simulink subsystem "PvtSubSys_LONC"  (R2020b)
settings: Solver=VariableStepAuto  StartTime=0.0  StopTime=10.0  RelTol=1e-3
undefined symbols (not defined in the file): P_Global_TireRadius_m, P_Global_Weight_N, P_LongCtrl_VLC_fRollCoef, P_LongCtrl_VLC_WindArea, P_LongCtrl_VLCaccelMinHoldXAxis, P_LongCtrl_VLCaccelMinHoldYAxis, P_LongCtrl_VLCaXCDeadZoneProp_Y, P_LongCtrl_VLCaXCKiCtrlDevChar_Y, P_LongCtrl_VLCaxCtrlDevDeadZoneChar_Y, P_LongCtrl_VLCaxCtrlDevEC2DCMax, P_LongCtrl_VLCaxCtrlDevFastQuitDCMode, P_LongCtrl_VLCaxCtrlDevThresAddEC2DC, P_LongCtrl_VLCaxCtrlDevTresAddDC2EC, P_LongCtrl_VLCAxTarDtThreEnableI, P_LongCtrl_VLCaxvRoadSlopeDC4CharXAxis, P_LongCtrl_VLCaxvRoadSlopeDC4CharYAxis, P_LongCtrl_VLCAxvTracMinDC1FullFillXAxis, P_LongCtrl_VLCAxvTracMinDC1FullFillYAxis, P_LongCtrl_VLCcoefFXAxis, P_LongCtrl_VLCcoefFYAxis, P_LongCtrl_VLCcoefIFadeOut1Calc, P_LongCtrl_VLCcoefIFadeOut1Condition, P_LongCtrl_VLCcoefIFadeOut2Calc, P_LongCtrl_VLCcoefIFadeOut2Condition, P_LongCtrl_VLCcoefIFadeOut3Calc, P_LongCtrl_VLCcoefIFadeOut3Condition, P_LongCtrl_VLCCounterAxvTracMinTimeout, P_LongCtrl_VLCCounterDC2ECTorqDelay, P_LongCtrl_VLCCounterDrvOff2EC, P_LongCtrl_VLCdaxTarEC2DCMax, P_LongCtrl_VLCdriveOffAxUpLimXAxix, P_LongCtrl_VLCdriveOffAxUpLimYAxix, P_LongCtrl_VLCDtAxvRef2UpperBandDC5, P_LongCtrl_VLCIACompensionNeg, P_LongCtrl_VLCIACompensionPos, P_LongCtrl_VLCjerkHoldXAxis, P_LongCtrl_VLCjerkHoldYAxis, P_LongCtrl_VLCki, P_LongCtrl_VLCkp, P_LongCtrl_VLCks, P_LongCtrl_VLCTorqDiffThreAxvTracMinTimeout, P_LongCtrl_VLCTrTatioMax, P_LongCtrl_VLCTrTatioMin, P_LongCtrl_VLCVlcAccThresAxvTracMinTimeout
libraries: simulink x32
(part 1 of 2)
settings Model: Creator=GW00133806  LastModifiedBy=GW00119710

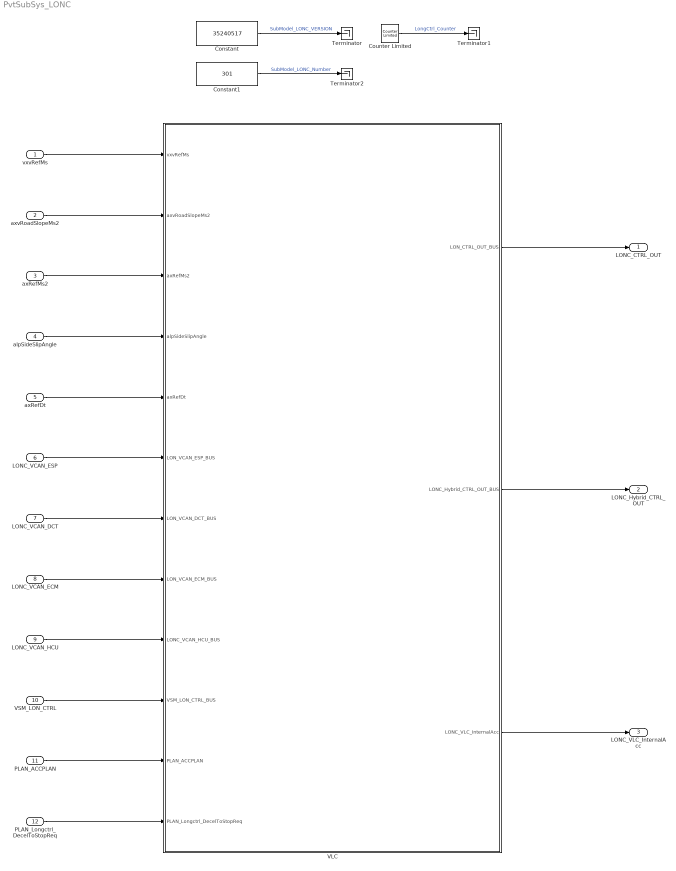
== system PvtSubSys_LONC ==
  vxvRefMs : Inport  OutDataTypeStr=single  PortDimensions=1  BusOutputAsStruct=on
  axvRoadSlopeMs2 : Inport  Port=2  OutDataTypeStr=single  PortDimensions=1  BusOutputAsStruct=on
  axRefMs2 : Inport  Port=3  OutDataTypeStr=single  PortDimensions=1  BusOutputAsStruct=on
  alpSideSlipAngle : Inport  Port=4  OutDataTypeStr=single  PortDimensions=1  BusOutputAsStruct=on
  axRefDt : Inport  Port=5  OutDataTypeStr=single  PortDimensions=1  BusOutputAsStruct=on
  LONC_VCAN_ESP : Inport  Port=6  OutDataTypeStr=Bus: VCAN_ESP_MSG_BUS  PortDimensions=1  BusOutputAsStruct=on
  LONC_VCAN_DCT : Inport  Port=7  OutDataTypeStr=Bus: VCAN_DCT_MSG_BUS  PortDimensions=1  BusOutputAsStruct=on
  LONC_VCAN_ECM : Inport  Port=8  OutDataTypeStr=Bus: VCAN_ECM_MSG_BUS  PortDimensions=1  BusOutputAsStruct=on
  LONC_VCAN_HCU : Inport  Port=9  OutDataTypeStr=Bus: VCAN_HCU_MSG_BUS  PortDimensions=1  BusOutputAsStruct=on
  VSM_LON_CTRL : Inport  Port=10  OutDataTypeStr=Bus: VSM_LON_CTRL_BUS  PortDimensions=1  BusOutputAsStruct=on
  PLAN_ACCPLAN : Inport  Port=11  OutDataTypeStr=Bus: PLAN_ACCPLAN_BUS
  PLAN_Longctrl_DecelToStopReq : Inport  Port=12  OutDataTypeStr=boolean  PortDimensions=1  BusOutputAsStruct=on
  Constant : Constant  Value=35240517  OutDataTypeStr=uint32
  Constant1 : Constant  Value=301  OutDataTypeStr=uint32
  Counter Limited : simulink/Sources/Counter Limited  uplimit=15  tsamp=-1
  Terminator : Terminator
  Terminator1 : Terminator
  Terminator2 : Terminator
  VLC : Subsystem
  LONC_CTRL_OUT : Outport  OutDataTypeStr=Bus: LONC_CTRL_OUT_BUS  PortDimensions=1  BusOutputAsStruct=on
  LONC_Hybrid_CTRL_OUT : Outport  Port=2  OutDataTypeStr=Bus: LONC_Hybrid_CTRL_OUT_BUS  PortDimensions=1  BusOutputAsStruct=on
  LONC_VLC_InternalAcc : Outport  Port=3  OutDataTypeStr=single
  wires:
  axRefDt/1 -> VLC/5(axRefDt)
  LONC_VCAN_ESP/1 -> VLC/6(LON_VCAN_ESP_BUS)
  PLAN_Longctrl_DecelToStopReq/1 -> VLC/12(PLAN_Longctrl_DecelToStopReq)
  alpSideSlipAngle/1 -> VLC/4(alpSideSlipAngle)
  vxvRefMs/1 -> VLC/1(vxvRefMs)
  Counter Limited/1 -> Terminator1/1  "LongCtrl_Counter"
  axRefMs2/1 -> VLC/3(axRefMs2)
  axvRoadSlopeMs2/1 -> VLC/2(axvRoadSlopeMs2)
  VLC/1(LON_CTRL_OUT_BUS) -> LONC_CTRL_OUT/1
  VSM_LON_CTRL/1 -> VLC/10(VSM_LON_CTRL_BUS)
  PLAN_ACCPLAN/1 -> VLC/11(PLAN_ACCPLAN)
  VLC/2(LONC_Hybrid_CTRL_OUT_BUS) -> LONC_Hybrid_CTRL_OUT/1
  LONC_VCAN_ECM/1 -> VLC/8(LON_VCAN_ECM_BUS)
  VLC/3(LONC_VLC_InternalAcc) -> LONC_VLC_InternalAcc/1
  LONC_VCAN_DCT/1 -> VLC/7(LON_VCAN_DCT_BUS)
  LONC_VCAN_HCU/1 -> VLC/9(LONC_VCAN_HCU_BUS)
  Constant/1 -> Terminator/1  "SubModel_LONC_VERSION"
  Constant1/1 -> Terminator2/1  "SubModel_LONC_Number"

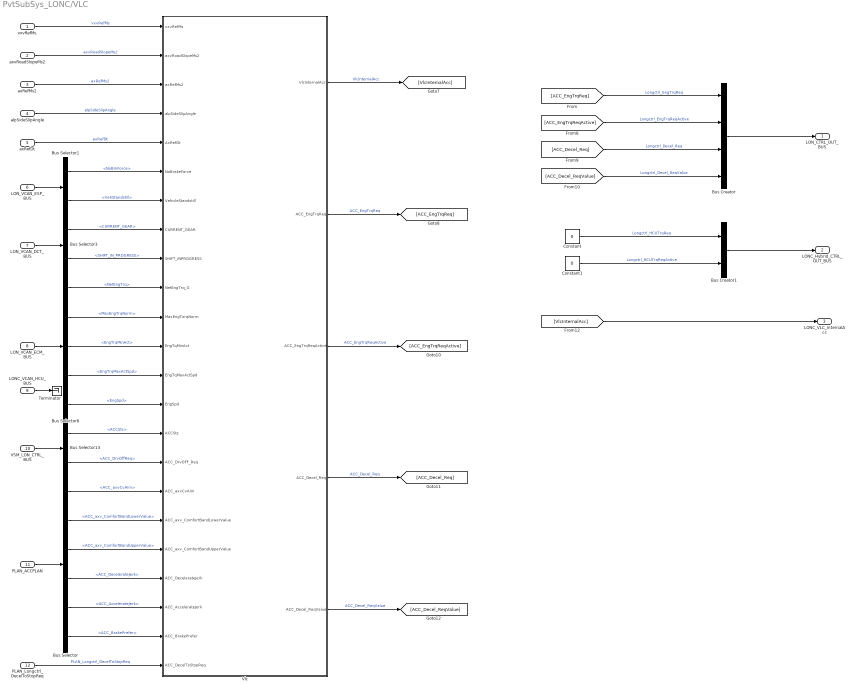
== system PvtSubSys_LONC/VLC ==
  vxvRefMs : Inport
  axvRoadSlopeMs2 : Inport  Port=2
  axRefMs2 : Inport  Port=3
  alpSideSlipAngle : Inport  Port=4
  axRefDt : Inport  Port=5
  LON_VCAN_ESP_BUS : Inport  Port=6  OutDataTypeStr=Bus: VCAN_ESP_MSG_BUS
  LON_VCAN_DCT_BUS : Inport  Port=7  OutDataTypeStr=Bus: VCAN_DCT_MSG_BUS
  LON_VCAN_ECM_BUS : Inport  Port=8  OutDataTypeStr=Bus: VCAN_ECM_MSG_BUS
  LONC_VCAN_HCU_BUS : Inport  Port=9  OutDataTypeStr=Bus: VCAN_HCU_MSG_BUS
  VSM_LON_CTRL_BUS : Inport  Port=10  OutDataTypeStr=Bus: VSM_LON_CTRL_BUS
  PLAN_ACCPLAN : Inport  Port=11  OutDataTypeStr=Bus: PLAN_ACCPLAN_BUS
  PLAN_Longctrl_DecelToStopReq : Inport  Port=12  OutDataTypeStr=boolean
  Bus Creator : BusCreator  Inputs=4  OutDataTypeStr=Bus: LONC_CTRL_OUT_BUS  NonVirtualBus=on
  Bus Creator1 : BusCreator  Inputs=2  OutDataTypeStr=Bus: LONC_Hybrid_CTRL_OUT_BUS  NonVirtualBus=on
  Bus Selector : BusSelector  OutputSignals=ACC_axvCvAim,ACC_axv_ComfortBandLowerValue,ACC_axv_ComfortBandUpperValue,ACC_DecelerateJerk,ACC_AccelerateJerk,ACC_BrakePrefer
  Bus Selector1 : BusSelector  OutputSignals=NoBrkForce,VehStandstill
  Bus Selector13 : BusSelector  OutputSignals=ACCSts,ACC_DrvOffReq
  Bus Selector3 : BusSelector  OutputSignals=CURRENT_GEAR,SHIFT_IN_PROGRESS
  Bus Selector6 : BusSelector  OutputSignals=NetEngTrq,MaxEngTrqNorm,EngTrqMinAct,EngTrqMaxActSpd,EngSpd
  Constant : Constant  Value=0  OutDataTypeStr=single
  Constant1 : Constant  Value=0  OutDataTypeStr=boolean
  Terminator : Terminator
  Vlc : Subsystem  TreatAsAtomicUnit=on
  LON_CTRL_OUT_BUS : Outport  OutDataTypeStr=Bus: LONC_CTRL_OUT_BUS
  LONC_Hybrid_CTRL_OUT_BUS : Outport  Port=2  OutDataTypeStr=Bus: LONC_Hybrid_CTRL_OUT_BUS
  LONC_VLC_InternalAcc : Outport  Port=3  OutDataTypeStr=single
  wires:
  LONC_VCAN_HCU_BUS/1 -> Terminator/1
  Constant/1 -> Bus Creator1/1  "Longctrl_HCUTrqReq"
  Constant1/1 -> Bus Creator1/2  "Longctrl_HCUTrqReqActive"
  Bus Creator1/1 -> LONC_Hybrid_CTRL_OUT_BUS/1
  PLAN_Longctrl_DecelToStopReq/1 -> Vlc/23(ACC_DecelToStopReq)  "PLAN_Longctrl_DecelToStopReq"
  [VlcInternalAcc] -> LONC_VLC_InternalAcc/1
  Bus Selector/1 -> Vlc/17(ACC_axvCvAim)  "<ACC_axvCvAim>"
  Bus Selector/6 -> Vlc/22(ACC_BrakePrefer)  "<ACC_BrakePrefer>"
  Bus Selector/2 -> Vlc/18(ACC_axv_ComfortBandLowerValue)  "<ACC_axv_ComfortBandLowerValue>"
  Bus Selector/3 -> Vlc/19(ACC_axv_ComfortBandUpperValue)  "<ACC_axv_ComfortBandUpperValue>"
  Bus Selector/5 -> Vlc/21(ACC_AccelerateJerk)  "<ACC_AccelerateJerk>"
  Bus Selector/4 -> Vlc/20(ACC_DecelerateJerk)  "<ACC_DecelerateJerk>"
  PLAN_ACCPLAN/1 -> Bus Selector/1
  alpSideSlipAngle/1 -> Vlc/4(alpSideSlipAngle)  "alpSideSlipAngle"
  Bus Selector13/2 -> Vlc/16(ACC_DrvOFF_Req)  "<ACC_DrvOffReq>"
  Bus Selector13/1 -> Vlc/15(ACCSts)  "<ACCSts>"
  VSM_LON_CTRL_BUS/1 -> Bus Selector13/1
  Bus Selector6/5 -> Vlc/14(EngSpd)  "<EngSpd>"
  Bus Selector6/4 -> Vlc/13(EngTqMaxActSpd)  "<EngTrqMaxActSpd>"
  Bus Selector6/3 -> Vlc/12(EngTqMinAct)  "<EngTrqMinAct>"
  Bus Selector6/2 -> Vlc/11(MaxEngTorqNorm)  "<MaxEngTrqNorm>"
  Bus Selector6/1 -> Vlc/10(NetEngTrq_G)  "<NetEngTrq>"
  LON_VCAN_ECM_BUS/1 -> Bus Selector6/1
  LON_VCAN_DCT_BUS/1 -> Bus Selector3/1
  Bus Selector3/2 -> Vlc/9(SHIFT_INPROGRESS)  "<SHIFT_IN_PROGRESS>"
  Bus Selector3/1 -> Vlc/8(CURRENT_GEAR)  "<CURRENT_GEAR>"
  LON_VCAN_ESP_BUS/1 -> Bus Selector1/1
  Bus Selector1/2 -> Vlc/7(VehicleStandstill)  "<VehStandstill>"
  Bus Selector1/1 -> Vlc/6(NoBrakeForce)  "<NoBrkForce>"
  axRefDt/1 -> Vlc/5(AxRefDt)  "axRefDt"
  axRefMs2/1 -> Vlc/3(axRefMs2)  "axRefMs2"
  axvRoadSlopeMs2/1 -> Vlc/2(axvRoadSlopeMs2)  "axvRoadSlopeMs2"
  vxvRefMs/1 -> Vlc/1(vxvRefMs)  "vxvRefMs"
  [ACC_EngTrqReqActive] -> Bus Creator/2  "Longctrl_EngTrqReqActive"
  Vlc/2(ACC_EngTrqReq) -> [ACC_EngTrqReq]  "ACC_EngTrqReq"
  Vlc/4(ACC_Decel_Req) -> [ACC_Decel_Req]  "ACC_Decel_Req"
  Vlc/1(VlcInternalAcc) -> [VlcInternalAcc]  "VlcInternalAcc"
  Vlc/5(ACC_Decel_ReqValue) -> [ACC_Decel_ReqValue]  "ACC_Decel_ReqValue"
  Vlc/3(ACC_EngTrqReqActive) -> [ACC_EngTrqReqActive]  "ACC_EngTrqReqActive"
  Bus Creator/1 -> LON_CTRL_OUT_BUS/1
  [ACC_Decel_Req] -> Bus Creator/3  "Longctrl_Decel_Req"
  [ACC_Decel_ReqValue] -> Bus Creator/4  "Longctrl_Decel_ReqValue"
  [ACC_EngTrqReq] -> Bus Creator/1  "Longctrl_EngTrqReq"

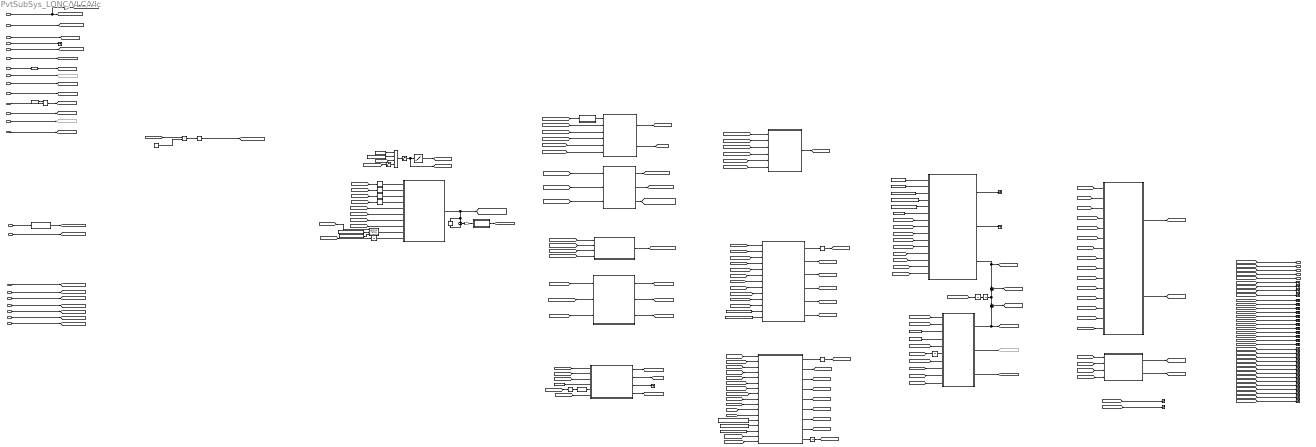
== system PvtSubSys_LONC/VLC/Vlc ==
  vxvRefMs : Inport  OutDataTypeStr=single
  axvRoadSlopeMs2 : Inport  Port=2  OutDataTypeStr=single
  axRefMs2 : Inport  Port=3  OutDataTypeStr=single
  alpSideSlipAngle : Inport  Port=4  OutDataTypeStr=single
  AxRefDt : Inport  Port=5  OutDataTypeStr=single
  NoBrakeForce : Inport  Port=6  OutDataTypeStr=boolean
  VehicleStandstill : Inport  Port=7  OutDataTypeStr=uint8
  CURRENT_GEAR : Inport  Port=8  OutDataTypeStr=uint8
  SHIFT_INPROGRESS : Inport  Port=9  OutDataTypeStr=boolean
  NetEngTrq_G : Inport  Port=10  OutDataTypeStr=single
  MaxEngTorqNorm : Inport  Port=11  OutDataTypeStr=uint16
  EngTqMinAct : Inport  Port=12  OutDataTypeStr=single
  EngTqMaxActSpd : Inport  Port=13  OutDataTypeStr=single
  EngSpd : Inport  Port=14  OutDataTypeStr=single
  ACCSts : Inport  Port=15  OutDataTypeStr=uint8
  ACC_DrvOFF_Req : Inport  Port=16  OutDataTypeStr=boolean
  ACC_axvCvAim : Inport  Port=17
  ACC_axv_ComfortBandLowerValue : Inport  Port=18
  ACC_axv_ComfortBandUpperValue : Inport  Port=19
  ACC_DecelerateJerk : Inport  Port=20
  ACC_AccelerateJerk : Inport  Port=21
  ACC_BrakePrefer : Inport  Port=22
  ACC_DecelToStopReq : Inport  Port=23
  AxTarUplimit : simulink/Lookup Tables/Lookup Table Dynamic  LookUpMeth=Interpolation-Use End Values  OutDataType=fixdt('single')  OutScaling=[]  OutputDataTypeScalingMode=Specify via dialog  OutDataTypeStr=single  DoSatur=off
  Compare To Constant8 : simulink/Logic and Bit Operations/Compare To Constant  relop===  const=1  OutDataTypeStr=boolean
  Compare To Zero : simulink/Logic and Bit Operations/Compare To Zero  relop===  OutDataTypeStr=boolean
  Constant : Constant  OutDataTypeStr=single
  Constant1 : Constant  Value=P_LongCtrl_VLCdriveOffAxUpLimYAxix  OutDataTypeStr=single
  Constant10 : Constant  Value=P_LongCtrl_VLCaxCtrlDevFastQuitDCMode  OutDataTypeStr=single
  Constant11 : Constant  Value=P_LongCtrl_VLCaxCtrlDevThresAddEC2DC  OutDataTypeStr=single
  Constant12 : Constant  Value=P_LongCtrl_VLCaxCtrlDevEC2DCMax  OutDataTypeStr=single
  Constant13 : Constant  Value=P_LongCtrl_VLCdaxTarEC2DCMax  OutDataTypeStr=single
  Constant2 : Constant  Value=P_LongCtrl_VLCkp  OutDataTypeStr=single
  Constant3 : Constant  Value=P_LongCtrl_VLCdriveOffAxUpLimXAxix  OutDataTypeStr=single
  Constant4 : Constant  Value=P_LongCtrl_VLCki  OutDataTypeStr=single
  Constant5 : Constant  Value=P_LongCtrl_VLCaXCDeadZoneProp_Y  OutDataTypeStr=single
  Constant8 : Constant  Value=10  OutDataTypeStr=single
  Constant9 : Constant  Value=P_LongCtrl_VLCaxCtrlDevTresAddDC2EC  OutDataTypeStr=single
  DC : Subsystem
  Data Type Conversion : DataTypeConversion  OutDataTypeStr=single
  EC : Subsystem
  FF_Control : Subsystem
  FxvCompensate : Constant  Value=0  OutDataTypeStr=single
  Gain1 : Gain  Gain=3.6  ParamDataTypeStr=single
  Gain2 : Gain  Gain=50
  Goto : Goto  Commented=on  GotoTag=CAN_Gear
  Goto26 : Goto  Commented=on  GotoTag=FFShiftInput
  Goto8 : Goto  Commented=on  GotoTag=CAN_EngTqMaxAct
  Ks : Constant  Value=P_LongCtrl_VLCks  OutDataTypeStr=single
  L  P : Subsystem
  L  P1 : Subsystem
  Ma_Ratio : Lookup_n-D  NumberOfTableDimensions=1  BreakpointsForDimension1=[3.38431,4.45086,5.42452,6.14307,6.90785,7.67253,8.43716,8.99323,9.82728,11.0319,12.0047,12.9774,13.8804,14.8066,15.6401,16.404,18,20]  Table=[1.04928,1.05921,1.07148,1.0827,1.09735,1.1143,1.1324,1.14598,1.1675,1.20037,1.23103,1.26514,1.29928,1.33456,1.36872,1.40176,1.41,1.41]  RndMeth=Simplest  InputSameDT=on
  Memory5 : Memory  InheritSampleTime=on
  Memory6 : Memory  InheritSampleTime=on
  Memory7 : Memory  InheritSampleTime=on
  MinMax1 : MinMax  Function=max  Inputs=2  OutDataTypeStr=single
  PI_Control : Subsystem
  PVLCaXCKiCtrlDevChar_Y : Constant  Value=P_LongCtrl_VLCaXCKiCtrlDevChar_Y  OutDataTypeStr=single
  P_VlcAxCtrlDevDeadZoneChar_Y : Constant  Value=P_LongCtrl_VLCaxCtrlDevDeadZoneChar_Y  OutDataTypeStr=single
  Product : Product  OutDataTypeStr=single
  Product5 : Product  Inputs=***/  RndMeth=Zero
  Saturation1 : Saturate  UpperLimit=180  LowerLimit=1.08
  Saturation2 : Saturate  UpperLimit=P_LongCtrl_VLCTrTatioMax  LowerLimit=P_LongCtrl_VLCTrTatioMin
  Subsystem : Subsystem
  Sum1 : Sum
  Sum2 : Sum
  Sum8 : Sum  Inputs=+-
  SwitchToBrakeMode : Subsystem
  SwitchToDriveMode : Subsystem
  Tapped Delay{2..5} (4 alike) : simulink/Discrete/Tapped Delay  vinit=0.0  samptime=-1  NumDelays=1  DelayOrder=Newest  includeCurrent=on
  Terminator{,5..23,25..37,45..46,48} (36 alike) : Terminator
  Trigonometric Function : Trigonometry  Operator=asin
  Unit Delay{,1..4} (5 alike) : UnitDelay  SampleTime=-1  HasFrameUpgradeWarning=on
  UpdateFlagCalc : Subsystem
  VLC_control_sts : Stateflow chart  TreatAsAtomicUnit=on
  VlcInternalAccCalc : MATLAB Function  TreatAsAtomicUnit=on
  VlcInternalFail : Constant  Value=0  OutDataTypeStr=uint8
  Weight/N1 : Constant  Value=0.377  OutDataTypeStr=single
  Weight/N2 : Constant  Value=P_Global_TireRadius_m
  axvClosedLoopControlCalc : Subsystem
  axvModelResidualCalc : Subsystem
  axvTracActMean_calc : Subsystem
  axvTracMin_calc : Subsystem
  g : Constant  Value=1/10  OutDataTypeStr=single
  VlcInternalAcc : Outport
  ACC_EngTrqReq : Outport  Port=2
  ACC_EngTrqReqActive : Outport  Port=3
  ACC_Decel_Req : Outport  Port=4
  ACC_Decel_ReqValue : Outport  Port=5
  wires:
  ACCSts/1 -> Subsystem/1(u)  "ACCSts"
  [ACC_DecelToStopReq] -> SwitchToDriveMode/11(StopReq)
  [VehSts_axvRoadSlope] -> DC/4(axvRoadSlopeMs2)
  SwitchToBrakeMode/4(Swit2DC_3) -> [SwDC_3]
  [VehSts_axvRoadSlope] -> SwitchToBrakeMode/4(axvRoadSlope)
  [CAN_ShiftInProgress] -> SwitchToBrakeMode/9("ShiftInProgress ")
  Constant12/1 -> SwitchToBrakeMode/14(P_VlcAxCtrlDevEC2DCMax)
  [AxRef_ms2] -> SwitchToBrakeMode/11(axRef)
  [ACCSts_ACCModeSts] -> SwitchToBrakeMode/7(ACC_Mode)
  [ACC_DecelToStopReq] -> SwitchToBrakeMode/6(StopReq)
  Memory6/1 -> [SwDC]
  SwitchToBrakeMode/6(Swit2DC_5) -> [SwDC_5]
  [axvTracMin] -> SwitchToBrakeMode/2(axvTracMin)
  SwitchToBrakeMode/9(Override2DC) -> Unit Delay2/1
  [ACC_BrakePrefer] -> SwitchToBrakeMode/10(BrakePrefer)
  SwitchToBrakeMode/3(Swit2DC_2) -> [SwDC_2]
  Constant11/1 -> SwitchToBrakeMode/13(P_VlcAxCtrlDevThresAddEC2DC)
  SwitchToBrakeMode/2(Swit2DC_1) -> [SwDC_1]
  SwitchToBrakeMode/1(SwitchToBrakeMode) -> Memory6/1
  SwitchToBrakeMode/5(Swit2DC_4) -> [SwDC_4]
  [VlcAxTarDt] -> SwitchToBrakeMode/12(VlcAxTarDt)
  [VlcInternalAcc] -> SwitchToBrakeMode/5(VlcAxTar)
  Unit Delay2/1 -> [OverrideToDC]
  [ACC_axvCvAim] -> SwitchToBrakeMode/3(axvCvAim)
  [ACC_axvComfortBandUpperValue] -> SwitchToBrakeMode/8(axv_ComfortBandUpperValue)
  SwitchToBrakeMode/7(Swit2DC_6) -> [SwDC_6]
  [VehSts_VxvRef_ms] -> SwitchToBrakeMode/1(VxvRef_ms)
  [CAN_NetEngTrq] -> SwitchToBrakeMode/17(CAN_NetEngTrq)
  [ACC_EngTorqReq] -> SwitchToBrakeMode/16(ACC_EngTorqReq)
  SwitchToBrakeMode/8(Swit2DC_7) -> [SwDC_7]
  Constant13/1 -> SwitchToBrakeMode/15(P_VlcdAxTarEC2DCMax)
  Tapped Delay3/1 -> VlcInternalAccCalc/2(DC)
  Tapped Delay5/1 -> VlcInternalAccCalc/4(ACC_Mode)
  [UpdateEnable_axvModeldiff] -> Terminator37/1  "LongCtrl_UpdateEnable_axvModeldiff"
  [FF_NetEngTorqMax] -> Terminator31/1  "LongCtrl_FF_NetEngTorqMax"
  alpSideSlipAngle/1 -> Terminator48/1  "Longctrl_VIE_alpSideSlipAngle"
  Trigonometric Function/1 -> [VehSts_SlopeAngle_rad]
  g/1 -> Product/2
  [VehSts_axvRoadSlope] -> Product/1
  axRefMs2/1 -> [AxRef_ms2]  "Longctrl_VIE_axRefMs2"
  Unit Delay1/1 -> VlcInternalAccCalc/10(VlcInternalAccK1)
  AxTarUplimit/1 -> VlcInternalAccCalc/9(DriveOffAxUpLim)
  PI_Control/3(PI_NetEngTorq) -> [PI_NetEngTorqInc], Sum1/1  "PI_NetEngTorq"
  [axvClosedLoopControl] -> FF_Control/1(AxTar)
  [Ma_Ratio] -> axvTracMin_calc/5(Ma)
  [PI_NetEngTorqInc] -> EC/14(PI_NetEngTorqInc)
  [ACCSts_ACCModeSts] -> VLC_control_sts/3(ACC_Mode)
  [VehSts_VxvRef_ms] -> AxTarUplimit/1
  [VehSts_VxvRef_kmh] -> axvTracMin_calc/3(VehicleSpd_kmh)
  Saturation1/1 -> Product5/4
  SwitchToDriveMode/1(SwitchToDriveMode) -> Memory7/1
  axvClosedLoopControlCalc/2(tauFxvCvFilter) -> [tauFxvCvFilter]
  [CAN_NetEngTrq] -> L  P1/1(Raw)
  [VehSts_VxvRef_ms] -> FF_Control/5(VxvRef_ms)
  [ACC_axvComfortBandLowerValue] -> SwitchToDriveMode/9(axv_ComfortBandLowerValue)
  [CAN_NoBrakeForce] -> UpdateFlagCalc/1(NoBrakeForce)
  [CAN_MaxEngTrq] -> axvTracActMean_calc/2(MaxEngTorq)
  [CAN_EngSpd] -> Product5/3
  Weight/N2/1 -> Product5/2
  Constant9/1 -> SwitchToDriveMode/12(P_VlcAxCtrlDevTresAddDC2EC)
  EC/2(Signal_ACC_EngTrqReqActive) -> [ACC_EngTorqReqActive]  "Signal_ACC_EngTrqReqActive"
  axvClosedLoopControlCalc/1(axvClosedLoopControl) -> [axvClosedLoopControl]
  [ACC_UpperJerk] -> EC/4(Accelerate_jerk)
  [ECEnable] -> PI_Control/10(ECEnable)
  [VehSts_VxvRef_kmh] -> PI_Control/9(Vego_kmh)
  [Tr_Ratio] -> axvTracActMean_calc/6(Tr)
  [CAN_ShiftInProgress] -> EC/11(ShiftInProgress)
  [CAN_ShiftInProgress] -> UpdateFlagCalc/2(DCT_ShiftInProgress)
  [tauFxvCvFilter] -> FF_Control/10(tauFxvCvFilter)
  [UpdateEnable_axvModeldiff] -> axvModelResidualCalc/2(Enable)
  [Tr_Ratio] -> axvTracMin_calc/6(Tr)
  PI_Control/1(Diff_grad) -> Terminator45/1
  [CAN_MaxEngTrq] -> axvTracMin_calc/2(MaxEngTorq)
  [Ma_Ratio] -> axvTracActMean_calc/5(Ma)
  VLC_control_sts/2(tEC) -> [tEC]
  [ACCSts_ACCModeSts] -> DC/3(ACCmode)
  [Tr_Ratio] -> FF_Control/8(Tr_Ratio)
  [ACC_BrakePrefer] -> SwitchToDriveMode/10(BrakePrefer)
  EC/1(ACC_EngTorqReq) -> [ACC_EngTorqReq]  "Signal_ACC_EngTrqReq"
  Unit Delay3/1 -> Unit Delay4/1
  Constant3/1 -> AxTarUplimit/2
  Weight/N1/1 -> Product5/1
  [ACC_axvCvAim] -> SwitchToDriveMode/8(AxvCvAim)
  [VlcInternalAcc] -> axvClosedLoopControlCalc/2(VlcInternalAcc)
  [VehSts_VxvRef_ms] -> EC/5(VxvRef_ms)
  Constant2/1 -> PI_Control/1(P_Gain)
  [axvDiff] -> PI_Control/8(axvDiff)
  [ACC_LowerJerk] -> EC/6(Decelerate_jerk)
  [AxRef_ms2] -> axvClosedLoopControlCalc/3(AxRef)
  [axvModelResidual] -> axvClosedLoopControlCalc/1(axvModelResidual)
  [ACC_LowerJerk] -> VlcInternalAccCalc/8(DeceJerk)
  [ACCSts_ACCModeSts] -> Tapped Delay5/1
  Compare To Zero/1 -> Data Type Conversion/1
  Sum8/1 -> Gain2/1
  axvClosedLoopControlCalc/3(Diff) -> [axvDiff]
  [FF_EngTorqInc] -> EC/13(FF_EngTorqInc)
  [AxRef_ms2] -> PI_Control/13(axvRef)
  [VlcInternalAcc] -> Unit Delay1/1
  Unit Delay4/1 -> Sum1/2, Sum2/1
  VlcInternalAccCalc/1(VlcInternalAcc) -> [VlcInternalAcc], Sum8/1, Memory5/1
  [VehSts_SlopeAngle_rad] -> axvTracActMean_calc/4(SlopeAngle_rad)
  [VehSts_VxvRef_kmh] -> axvTracActMean_calc/3(VehicleSpd_kmh)
  [tEC] -> EC/3(tEC)
  UpdateFlagCalc/1(UpdateEnable) -> [UpdateEnable_axvModeldiff]
  VLC_control_sts/3(tDC) -> Terminator/1
  SwitchToDriveMode/6(Swit2EC_5) -> [SwEC_5]
  L  P1/1(Out) -> axvTracActMean_calc/1(Torq)
  [CAN_MaxEngTrq] -> EC/10(MaxEngTrq)
  L  P/1(Out) -> [VlcAxTarDt]
  axvTracActMean_calc/1(axvTracActMean) -> [axvTracActMean]
  [CAN_MaxEngTrq] -> FF_Control/7(MaxEngTrq)
  SwitchToDriveMode/4(Swit2EC_3) -> [SwEC_3]
  [ACCSts_DriveOffReq] -> Tapped Delay4/1
  [AxRef_ms2] -> SwitchToDriveMode/5(axRef)
  [CAN_ShiftInProgress] -> PI_Control/15(ShiftInProgress)
  PI_Control/2(BigDeadzoneValue) -> Terminator46/1
  [ACC_axvCvAim] -> VlcInternalAccCalc/6(AxTar)
  axvModelResidualCalc/3(axvModelResidual) -> [axvModelResidual]
  Data Type Conversion/1 -> VLC_control_sts/5(Motorial)
  [CAN_EngSpd] -> EC/2(EngSpd)
  [VehSts_SlopeAngle_rad] -> axvTracMin_calc/4(SlopeAngle_rad)
  [VlcInternalAcc] -> DC/2(VlcAxTar)
  [DCEnable] -> DC/1(DC_enable)
  [AxRef_ms2] -> axvModelResidualCalc/1(AxRef)
  Memory7/1 -> [SwEC]
  [AxRef_ms2] -> VlcInternalAccCalc/5(AxRef)
  Sum2/1 -> [FF_NetEngTorq]
  Ma_Ratio/1 -> [Ma_Ratio]
  Saturation2/1 -> Ma_Ratio/1, [Tr_Ratio]
  [Fz] -> FF_Control/2(Fz)
  Constant5/1 -> PI_Control/3(P_VlcAXCDeadZoneProp_Y)
  Sum1/1 -> [PI_NetEngTorq]
  DC/2(ACC_Decel_ReqValue) -> [ACC_DecelReqValue]  "Signal_ACC_Decel_ReqValue"
  [ACCSts_ACCModeSts] -> SwitchToDriveMode/1(ACC_Mode)
  [SwEC] -> VLC_control_sts/1(SwitchToDriveMode)
  [VlcInternalAcc] -> SwitchToDriveMode/6(VlcAxTar)
  axvTracMin_calc/1(axvTracMin) -> [axvTracMin]
  [ECEnable] -> EC/1(ECEnable)
  VLC_control_sts/4(DCEnable) -> [DCEnable]
  [CAN_MaxEngTrq] -> PI_Control/12(MaxEngTrq)
  [Tr_Ratio] -> PI_Control/11(Tr_Ratio)
  [VehSts_VxvRef_kmh] -> Saturation1/1
  P_VlcAxCtrlDevDeadZoneChar_Y/1 -> PI_Control/4(P_VlcAxCtrlDevDeadZoneChar_Y)
  axvModelResidualCalc/2(axvModel_Ref) -> [axvModelRef]
  FF_Control/3(FF_NetEngTorqMax) -> [FF_NetEngTorqMax]
  FF_Control/1(FF_NetEngTorqInc) -> [FF_EngTorqInc], Sum2/2
  [SwDC] -> VLC_control_sts/2(SwitchToBrakeMode)
  [CAN_EngTqMinAct] -> axvTracMin_calc/1(Torq)
  FF_Control/2(FFShiftInput) -> Goto26/1
  axvTracActMean_calc/2(Fz) -> [Fz]
  [OverrideToDC] -> VLC_control_sts/6(OverrideToDC)
  SwitchToDriveMode/2(Swit2EC_1) -> [SwEC_1]
  Unit Delay/1 -> FF_Control/6(ACC_EngTorqReqK1)
  [CAN_NetEngTrq] -> EC/12(NetEngTrq)
  SwitchToDriveMode/5(Swit2EC_4) -> [SwEC_4]
  Memory5/1 -> Sum8/2
  [ACCSts_VehStandstill] -> Compare To Zero/1
  Tapped Delay2/1 -> VlcInternalAccCalc/1(EC)
  PVLCaXCKiCtrlDevChar_Y/1 -> PI_Control/5(P_VlcAXCKiCtrlDevChar_Y)
  [ACC_UpperJerk] -> VlcInternalAccCalc/7(AcceJerk)
  VlcInternalFail/1 -> VLC_control_sts/4(VLCInternalFailSts)
  DC/1(ACC_Decel_Req) -> [ACC_DecelReq]  "Signal_ACC_Decel_Req"
  [VehSts_axvRoadSlope] -> SwitchToDriveMode/4(AxvRoadSlope)
  Gain2/1 -> L  P/1(Raw)
  [DCEnable] -> Tapped Delay3/1
  axvModelResidualCalc/1(axvModeldiff) -> [axvModeldiff]
  [axvTracActMean] -> axvModelResidualCalc/3(axvTorqMean)
  [CAN_NoBrakeForce] -> SwitchToDriveMode/3(NoBrakeForce)
  [Ma_Ratio] -> EC/8(Ma_Ratio)
  [VlcAxTarDt] -> SwitchToDriveMode/7(VlcAxTarDt)
  [DCEnable] -> EC/7(DCEnable)
  FxvCompensate/1 -> FF_Control/4(FxvCompensate)
  Product5/1 -> Saturation2/1
  SwitchToDriveMode/3(Swit2EC_2) -> [SwEC_2]
  [VlcAxTarDt] -> PI_Control/7(VlcAxTarDt)
  [ACC_EngTorqReq] -> Unit Delay/1
  Constant10/1 -> SwitchToDriveMode/13(P_VlcAxCtrlDevFastQuitDCMode)
  [VlcInternalAcc] -> PI_Control/14(GetVlcAxTar)
  [VehSts_AxRefDt] -> UpdateFlagCalc/3(AxRefDt)
  [VehSts_VxvRef_kmh] -> UpdateFlagCalc/4(Vxv)
  [ACCSts_DriveOffReq] -> EC/15(DiveOff)
  [Ma_Ratio] -> FF_Control/9(Ma_Ratio)
  [CAN_NetEngTrq] -> Unit Delay3/1
  [ECEnable] -> Tapped Delay2/1
  Constant8/1 -> PI_Control/6(P_VlcWindupLim)
  [ACCSts_DriveOffReq] -> SwitchToDriveMode/2(DriveOff)
  Tapped Delay4/1 -> VlcInternalAccCalc/3(DriveOff)
  Ks/1 -> FF_Control/3(Ks_Gain)
  Constant1/1 -> AxTarUplimit/3
  VLC_control_sts/1(ECEnable) -> [ECEnable]
  Constant4/1 -> PI_Control/2(I_Gain)
  [Tr_Ratio] -> EC/9(Tr_Ratio)
  [SwDC_4] -> Terminator21/1  "LongCtrl_Sw2DC4"
  [SwEC] -> Terminator33/1  "LongCtrl_Sw2EC"
  [Fz] -> Terminator9/1  "LongCtrl_Fz"
  [SwDC_5] -> Terminator22/1  "LongCtrl_Sw2DC5"
  [axvModelRef] -> Terminator15/1  "LongCtrl_axvModelRef"
  [SwDC] -> Terminator25/1  "LongCtrl_Sw2DC"
  [ACC_DecelReq] -> ACC_Decel_Req/1  "LongCtrl_ACC_Decel_Req"
  [axvModeldiff] -> Terminator20/1  "LongCtrl_axvModelDiff"
  [axvDiff] -> Terminator17/1  "LongCtrl_axvDiff"
  [OverrideToDC] -> Terminator12/1  "LongCtrl_OverrideToDC"
  [FF_EngTorqInc] -> Terminator8/1  "LongCtrl_FF_NetEngTorqInc"
  [axvClosedLoopControl] -> Terminator16/1  "LongCtrl_axvClosedLoopControl"
  [PI_NetEngTorqInc] -> Terminator6/1  "LongCtrl_PI_NetEngTorqInc"
  [VlcInternalAcc] -> VlcInternalAcc/1  "LongCtrl_VlcInternalAcc"
  [SwDC_7] -> Terminator32/1  "LongCtrl_Sw2DC7"
  [SwDC_3] -> Terminator28/1  "LongCtrl_Sw2DC3"
  [axvTracActMean] -> Terminator19/1  "LongCtrl_axvTracActMean"
  [FF_NetEngTorq] -> Terminator7/1  "LongCtrl_FF_NetEngTorq"
  [SwEC_3] -> Terminator36/1  "LongCtrl_Sw2EC3"
  [DCEnable] -> Terminator11/1  "LongCtrl_DCEnable"
  [SwDC_1] -> Terminator26/1  "LongCtrl_Sw2DC1"
  [SwEC_4] -> Terminator29/1  "LongCtrl_Sw2EC4"
  [Tr_Ratio] -> Terminator14/1  "LongCtrl_Tr_Ratio"
  [ECEnable] -> Terminator10/1  "LongCtrl_ECEnable"
  [ACC_DecelReqValue] -> ACC_Decel_ReqValue/1  "LongCtrl_ACC_Decel_ReqValue"
  [axvTracMin] -> Terminator13/1  "LongCtrl_axvTracMin"
  [SwEC_5] -> Terminator30/1  "LongCtrl_Sw2EC5"
  [SwEC_2] -> Terminator35/1  "LongCtrl_Sw2EC2"
  [ACC_EngTorqReq] -> ACC_EngTrqReq/1  "LongCtrl_ACC_EngTrqReq"
  [SwDC_6] -> Terminator23/1  "LongCtrl_Sw2DC6"
  [PI_NetEngTorq] -> Terminator5/1  "LongCtrl_PI_NetEngTorq"
  [axvModelResidual] -> Terminator18/1  "LongCtrl_axvModelResidual"
  [SwEC_1] -> Terminator34/1  "LongCtrl_Sw2EC1"
  [ACC_EngTorqReqActive] -> ACC_EngTrqReqActive/1  "LongCtrl_ACC_EngTrqReqActive"
  [SwDC_2] -> Terminator27/1  "LongCtrl_Sw2DC2"
  Compare To Constant8/1 -> [ACCSts_VehStandstill]
  VehicleStandstill/1 -> Compare To Constant8/1
  SHIFT_INPROGRESS/1 -> [CAN_ShiftInProgress]
  Subsystem/1(ACCModeSts) -> [ACCSts_ACCModeSts]  "ACCSts"
  NetEngTrq_G/1 -> [CAN_NetEngTrq]
  NoBrakeForce/1 -> [CAN_NoBrakeForce]
  axvRoadSlopeMs2/1 -> [VehSts_axvRoadSlope]  "axvRoadSlopeMs2"
  ACC_DecelToStopReq/1 -> [ACC_DecelToStopReq]
  ACC_axvCvAim/1 -> [ACC_axvCvAim]
  Gain1/1 -> [VehSts_VxvRef_kmh]
  CURRENT_GEAR/1 -> Goto/1
  EngTqMaxActSpd/1 -> Goto8/1
  MinMax1/1 -> [CAN_MaxEngTrq]
  ACC_BrakePrefer/1 -> [ACC_BrakePrefer]
  ACC_DecelerateJerk/1 -> [ACC_LowerJerk]
  EngSpd/1 -> [CAN_EngSpd]
  MaxEngTorqNorm/1 -> MinMax1/2
  vxvRefMs/1 -> [VehSts_VxvRef_ms], Gain1/1  "vxvRefMs"
  ACC_DrvOFF_Req/1 -> [ACCSts_DriveOffReq]  "ACC_DrvOFF_Req"
  Product/1 -> Trigonometric Function/1
  ACC_AccelerateJerk/1 -> [ACC_UpperJerk]
  ACC_axv_ComfortBandUpperValue/1 -> [ACC_axvComfortBandUpperValue]
  ACC_axv_ComfortBandLowerValue/1 -> [ACC_axvComfortBandLowerValue]
  Constant/1 -> MinMax1/1
  AxRefDt/1 -> [VehSts_AxRefDt]  "Longctrl_VIE_AxRefDt"
  EngTqMinAct/1 -> [CAN_EngTqMinAct]

== system PvtSubSys_LONC/VLC/Vlc/DC ==
  DC_enable : Inport
  VlcAxTar : Inport  Port=2
  ACCmode : Inport  Port=3
  axvRoadSlopeMs2 : Inport  Port=4
  1-D Lookup Table : Lookup_n-D  NumberOfTableDimensions=1  BreakpointsForDimension1=P_LongCtrl_VLCaccelMinHoldXAxis  Table=P_LongCtrl_VLCaccelMinHoldYAxis  ExtrapMethod=Clip  InternalRulePriority=Speed  OutDataTypeStr=single  RndMeth=Simplest  InputSameDT=on
  1-D Lookup Table1 : Lookup_n-D  NumberOfTableDimensions=1  BreakpointsForDimension1=P_LongCtrl_VLCjerkHoldXAxis  Table=P_LongCtrl_VLCjerkHoldYAxis  ExtrapMethod=Clip  InternalRulePriority=Speed  OutDataTypeStr=single  RndMeth=Simplest  InputSameDT=on
  Logical Operator : Logic  Operator=OR  AllPortsSameDT=off  OutDataTypeStr=boolean
  Product1 : Product  RndMeth=Zero
  StandstillAccel2 : Stateflow chart  TreatAsAtomicUnit=on
  Tapped Delay : simulink/Discrete/Tapped Delay  vinit=0.0  samptime=-1  NumDelays=1  DelayOrder=Newest  includeCurrent=on
  ACC_Decel_Req : Outport
  ACC_Decel_ReqValue : Outport  Port=2
  wires:
  1-D Lookup Table1/1 -> StandstillAccel2/4(jerkHold)
  1-D Lookup Table/1 -> StandstillAccel2/3(accelHoldMin)
  axvRoadSlopeMs2/1 -> 1-D Lookup Table/1, 1-D Lookup Table1/1
  StandstillAccel2/2(decelReq) -> ACC_Decel_ReqValue/1
  ACCmode/1 -> Tapped Delay/1
  VlcAxTar/1 -> Product1/2
  DC_enable/1 -> Logical Operator/1, Product1/1
  Product1/1 -> StandstillAccel2/1(VlcAxTar)
  Tapped Delay/1 -> StandstillAccel2/2(ACCmode)
  StandstillAccel2/1(decelReqActive) -> Logical Operator/2
  Logical Operator/1 -> ACC_Decel_Req/1

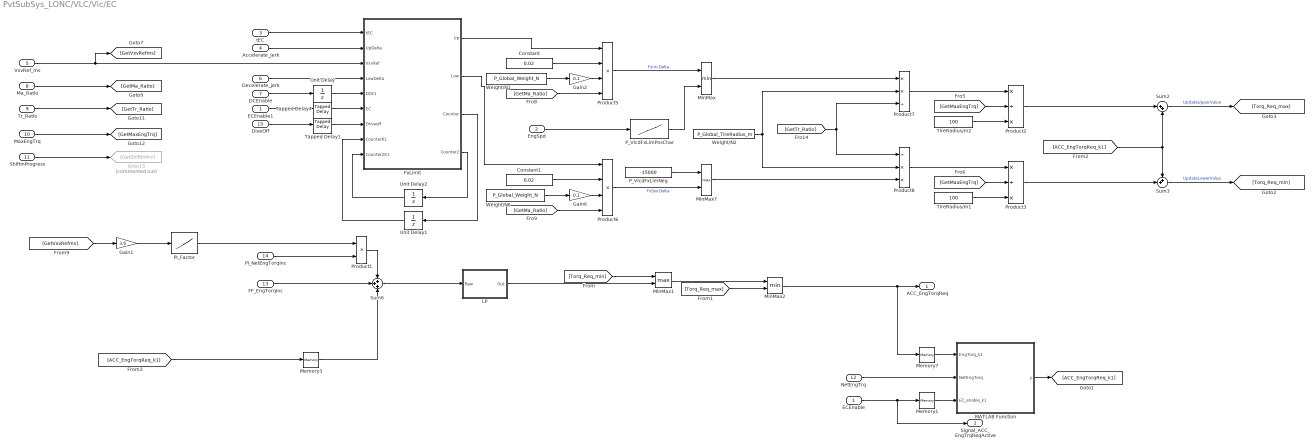
== system PvtSubSys_LONC/VLC/Vlc/EC ==
  ECEnable : Inport
  EngSpd : Inport  Port=2
  tEC : Inport  Port=3
  Accelerate_jerk : Inport  Port=4
  VxvRef_ms : Inport  Port=5
  Decelerate_jerk : Inport  Port=6
  DCEnable : Inport  Port=7
  Ma_Ratio : Inport  Port=8
  Tr_Ratio : Inport  Port=9
  MaxEngTrq : Inport  Port=10
  ShiftInProgress : Inport  Port=11
  NetEngTrq : Inport  Port=12
  FF_EngTorqInc : Inport  Port=13
  PI_NetEngTorqInc : Inport  Port=14
  DiveOff : Inport  Port=15  OutDataTypeStr=boolean
  Constant : Constant  Value=0.02  OutDataTypeStr=single
  Constant1 : Constant  Value=0.02  OutDataTypeStr=single
  ECEnable1 : InportShadow
  FxLimit : MATLAB Function  TreatAsAtomicUnit=on
  Gain1 : Gain  Gain=3.6
  Gain2 : Gain  Gain=0.1
  Gain6 : Gain  Gain=0.1
  Goto13 : Goto  Commented=on  GotoTag=GetShiftInPro
  LP : Subsystem
  MATLAB Function : MATLAB Function  TreatAsAtomicUnit=on
  Memory1 : Memory  InheritSampleTime=on
  Memory3 : Memory  InheritSampleTime=on
  Memory7 : Memory  InheritSampleTime=on
  MinMax : MinMax  Inputs=2
  MinMax1 : MinMax  Function=max  Inputs=2
  MinMax2 : MinMax  Inputs=2
  MinMax7 : MinMax  Function=max  Inputs=2
  "PI_Factor " : Lookup_n-D  NumberOfTableDimensions=1  BreakpointsForDimension1=[0,1.08,4,10]  Table=[0,0,1,1]  RndMeth=Simplest  InputSameDT=on
  P_VlcdFxLimNeg : Constant  Value=-15000  OutDataTypeStr=single
  "P_VlcdFxLimPosChar " : Lookup_n-D  NumberOfTableDimensions=1  BreakpointsForDimension1=[500,1000,1100]  Table=[1500,3000,10000]  RndMeth=Simplest  InputSameDT=on
  Product1 : Product  RndMeth=Zero
  Product2 : Product  Inputs=*/*  RndMeth=Zero
  Product3 : Product  Inputs=*/*  RndMeth=Zero
  Product5 : Product  Inputs=4  RndMeth=Zero
  Product6 : Product  Inputs=4  RndMeth=Zero
  Product7 : Product  Inputs=**/  RndMeth=Zero
  Product8 : Product  Inputs=/**  RndMeth=Zero
  Sum2 : Sum  Inputs=|++
  Sum3 : Sum  Inputs=++|
  Sum6 : Sum  Inputs=+++
  Tapped Delay1 : simulink/Discrete/Tapped Delay  vinit=0.0  samptime=-1  NumDelays=1  DelayOrder=Newest  includeCurrent=on
  Tapped Delay4 : simulink/Discrete/Tapped Delay  vinit=0.0  samptime=-1  NumDelays=1  DelayOrder=Newest  includeCurrent=on
  TireRadius/m1 : Constant  Value=100  OutDataTypeStr=single
  TireRadius/m2 : Constant  Value=100  OutDataTypeStr=single
  Unit Delay : UnitDelay  SampleTime=-1  HasFrameUpgradeWarning=on
  Unit Delay1 : UnitDelay  InitialCondition=single(0)  SampleTime=-1  HasFrameUpgradeWarning=on
  Unit Delay2 : UnitDelay  InitialCondition=single(0)  SampleTime=-1  HasFrameUpgradeWarning=on
  Weight/N1 : Constant  Value=P_Global_Weight_N  OutDataTypeStr=single
  Weight/N2 : Constant  Value=P_Global_TireRadius_m  OutDataTypeStr=single
  Weight/N6 : Constant  Value=P_Global_Weight_N  OutDataTypeStr=single
  ACC_EngTorqReq : Outport
  Signal_ACC_EngTrqReqActive : Outport  Port=2
  wires:
  Unit Delay2/1 -> FxLimit/9(Counter2K1)
  FxLimit/4(Counter2) -> Unit Delay2/1
  Unit Delay1/1 -> FxLimit/8(CounterK1)
  NetEngTrq/1 -> MATLAB Function/2(NetEngTorq)
  [Torq_Req_max] -> MinMax2/2
  MinMax1/1 -> MinMax2/1
  [Torq_Req_min] -> MinMax1/1
  LP/1(Out) -> MinMax1/2
  Sum2/1 -> [Torq_Req_max]  "UpdateUpperValue"
  [ACC_EngTorqReq_k1] -> Sum2/2, Sum3/1
  Product2/1 -> Sum2/1
  Sum3/1 -> [Torq_Req_min]  "UpdateLowerValue"
  Product3/1 -> Sum3/2
  DiveOff/1 -> Tapped Delay1/1
  Tapped Delay4/1 -> FxLimit/6(EC)
  Tapped Delay1/1 -> FxLimit/7(Driveoff)
  Unit Delay/1 -> FxLimit/5(DCK1)
  MaxEngTrq/1 -> [GetMaxEngTrq]
  ShiftInProgress/1 -> Goto13/1
  Tr_Ratio/1 -> [GetTr_Ratio]
  Ma_Ratio/1 -> [GetMa_Ratio]
  Memory3/1 -> Sum6/3
  [ACC_EngTorqReq_k1] -> Memory3/1
  FF_EngTorqInc/1 -> Sum6/2
  Gain1/1 -> "PI_Factor "/1
  [GetVxvRefms] -> Gain1/1
  MinMax2/1 -> Memory7/1, ACC_EngTorqReq/1
  VxvRef_ms/1 -> FxLimit/3(VxvRef), [GetVxvRefms]
  Sum6/1 -> LP/1(Raw)
  ECEnable1/1 -> Tapped Delay4/1
  FxLimit/3(Counter) -> Unit Delay1/1
  DCEnable/1 -> Unit Delay/1
  Product8/1 -> Product3/1
  [GetMaxEngTrq] -> Product3/2
  TireRadius/m1/1 -> Product3/3
  Product7/1 -> Product2/1
  [GetMaxEngTrq] -> Product2/2
  TireRadius/m2/1 -> Product2/3
  FxLimit/2(Low) -> Product6/1
  FxLimit/1(Up) -> Product5/1
  tEC/1 -> FxLimit/1(tEC)
  MinMax7/1 -> Product8/3
  [GetTr_Ratio] -> Product8/1, Product7/3
  Weight/N2/1 -> Product8/2, Product7/2
  MinMax/1 -> Product7/1
  [GetMa_Ratio] -> Product6/4
  Gain6/1 -> Product6/3
  Weight/N6/1 -> Gain6/1
  Constant1/1 -> Product6/2
  Decelerate_jerk/1 -> FxLimit/4(LowDelta)
  [GetMa_Ratio] -> Product5/4
  P_VlcdFxLimNeg/1 -> MinMax7/1
  Product6/1 -> MinMax7/2  "FxDecDelta"
  "P_VlcdFxLimPosChar "/1 -> MinMax/2
  EngSpd/1 -> "P_VlcdFxLimPosChar "/1
  Product5/1 -> MinMax/1  "FxIncDelta"
  Gain2/1 -> Product5/3
  Weight/N1/1 -> Gain2/1
  Constant/1 -> Product5/2
  Accelerate_jerk/1 -> FxLimit/2(UpDelta)
  Memory1/1 -> MATLAB Function/3(EC_enable_k1)
  ECEnable/1 -> Memory1/1, Signal_ACC_EngTrqReqActive/1
  Product1/1 -> Sum6/1
  "PI_Factor "/1 -> Product1/1
  PI_NetEngTorqInc/1 -> Product1/2
  MATLAB Function/1(y) -> [ACC_EngTorqReq_k1]
  Memory7/1 -> MATLAB Function/1(EngTorq_k1)

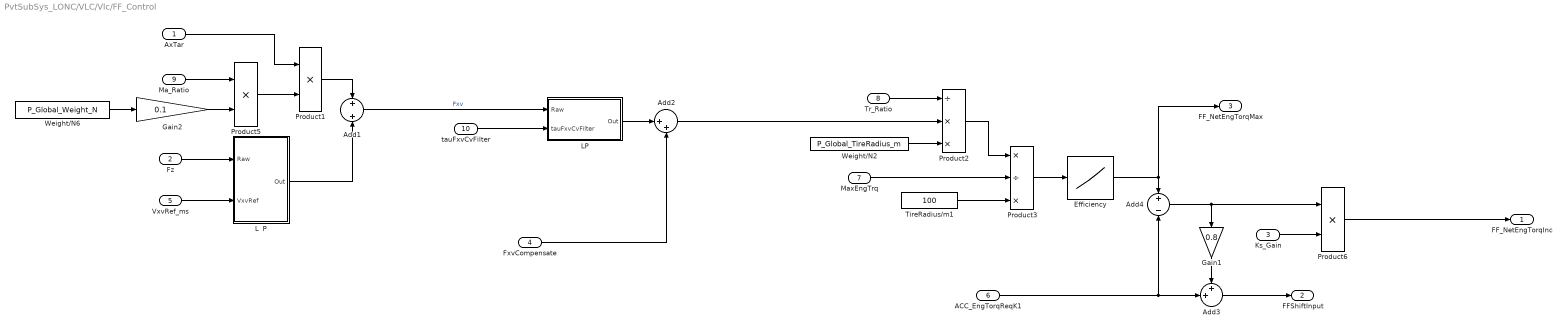
== system PvtSubSys_LONC/VLC/Vlc/FF_Control ==
  AxTar : Inport  OutDataTypeStr=single
  Fz : Inport  Port=2  OutDataTypeStr=single
  Ks_Gain : Inport  Port=3  OutDataTypeStr=single
  FxvCompensate : Inport  Port=4  OutDataTypeStr=single
  VxvRef_ms : Inport  Port=5  OutDataTypeStr=single
  ACC_EngTorqReqK1 : Inport  Port=6  OutDataTypeStr=single
  MaxEngTrq : Inport  Port=7  OutDataTypeStr=single
  Tr_Ratio : Inport  Port=8  OutDataTypeStr=single
  Ma_Ratio : Inport  Port=9  OutDataTypeStr=single
  tauFxvCvFilter : Inport  Port=10  OutDataTypeStr=single
  Add1 : Sum
  Add2 : Sum  Inputs=|++
  Add3 : Sum  Inputs=++|
  Add4 : Sum  Inputs=+-
  Efficiency : Lookup_n-D  NumberOfTableDimensions=1  BreakpointsForDimension1=[-110,-22,0,18,90]  Table=[-100,-20,0,20,100]  RndMeth=Simplest  InputSameDT=on
  Gain1 : Gain  Gain=0.8
  Gain2 : Gain  Gain=0.1
  L  P : Subsystem
  LP : Subsystem
  Product1 : Product  RndMeth=Zero
  Product2 : Product  Inputs=/**  RndMeth=Zero
  Product3 : Product  Inputs=*/*  RndMeth=Zero
  Product5 : Product  Inputs=**  RndMeth=Zero
  Product6 : Product  RndMeth=Zero
  TireRadius/m1 : Constant  Value=100  OutDataTypeStr=single
  Weight/N2 : Constant  Value=P_Global_TireRadius_m
  Weight/N6 : Constant  Value=P_Global_Weight_N
  FF_NetEngTorqInc : Outport  OutDataTypeStr=single
  FFShiftInput : Outport  Port=2  OutDataTypeStr=single
  FF_NetEngTorqMax : Outport  Port=3  OutDataTypeStr=single
  wires:
  tauFxvCvFilter/1 -> LP/2(tauFxvCvFilter)
  VxvRef_ms/1 -> L  P/2(VxvRef)
  L  P/1(Out) -> Add1/2
  Tr_Ratio/1 -> Product2/1
  Add3/1 -> FFShiftInput/1
  Gain1/1 -> Add3/1
  ACC_EngTorqReqK1/1 -> Add3/2, Add4/2
  FxvCompensate/1 -> Add2/2
  LP/1(Out) -> Add2/1
  Add4/1 -> Product6/1, Gain1/1
  Add2/1 -> Product2/2
  Add1/1 -> LP/1(Raw)  "Fxv"
  Product6/1 -> FF_NetEngTorqInc/1
  Ks_Gain/1 -> Product6/2
  AxTar/1 -> Product1/1
  Efficiency/1 -> Add4/1, FF_NetEngTorqMax/1
  Weight/N2/1 -> Product2/3
  Product1/1 -> Add1/1
  Fz/1 -> L  P/1(Raw)
  Product3/1 -> Efficiency/1
  Product2/1 -> Product3/1
  MaxEngTrq/1 -> Product3/2
  TireRadius/m1/1 -> Product3/3
  Weight/N6/1 -> Gain2/1
  Gain2/1 -> Product5/2
  Product5/1 -> Product1/2
  Ma_Ratio/1 -> Product5/1

== system PvtSubSys_LONC/VLC/Vlc/L  P ==
  Raw : Inport
  Constant2 : Constant  Value=0.02  OutDataTypeStr=single
  FilterTime1 : Constant  Value=0.1  OutDataTypeStr=single
  Product2 : Product  Inputs=*/  RndMeth=Zero
  Product6 : Product  RndMeth=Zero
  Sum6 : Sum  Inputs=+-  OutDataTypeStr=single
  Sum7 : Sum  OutDataTypeStr=single
  Unit Delay : UnitDelay  SampleTime=-1  HasFrameUpgradeWarning=on
  Out : Outport
  wires:
  Raw/1 -> Sum6/1
  Product6/1 -> Sum7/1
  Product2/1 -> Product6/1
  Sum6/1 -> Product6/2
  FilterTime1/1 -> Product2/2
  Constant2/1 -> Product2/1
  Unit Delay/1 -> Sum7/2, Sum6/2
  Sum7/1 -> Out/1, Unit Delay/1

== system PvtSubSys_LONC/VLC/Vlc/L  P1 ==
  Raw : Inport
  Constant2 : Constant  Value=0.02  OutDataTypeStr=single
  FilterTime1 : Constant  Value=0.1  OutDataTypeStr=single
  Memory4 : Memory  InheritSampleTime=on
  Product2 : Product  Inputs=*/  RndMeth=Zero
  Product6 : Product  RndMeth=Zero
  Sum6 : Sum  Inputs=+-
  Sum7 : Sum
  Out : Outport
  wires:
  Raw/1 -> Sum6/1
  Product6/1 -> Sum7/1
  Product2/1 -> Product6/1
  Sum6/1 -> Product6/2
  FilterTime1/1 -> Product2/2
  Constant2/1 -> Product2/1
  Memory4/1 -> Sum7/2, Sum6/2
  Sum7/1 -> Memory4/1, Out/1

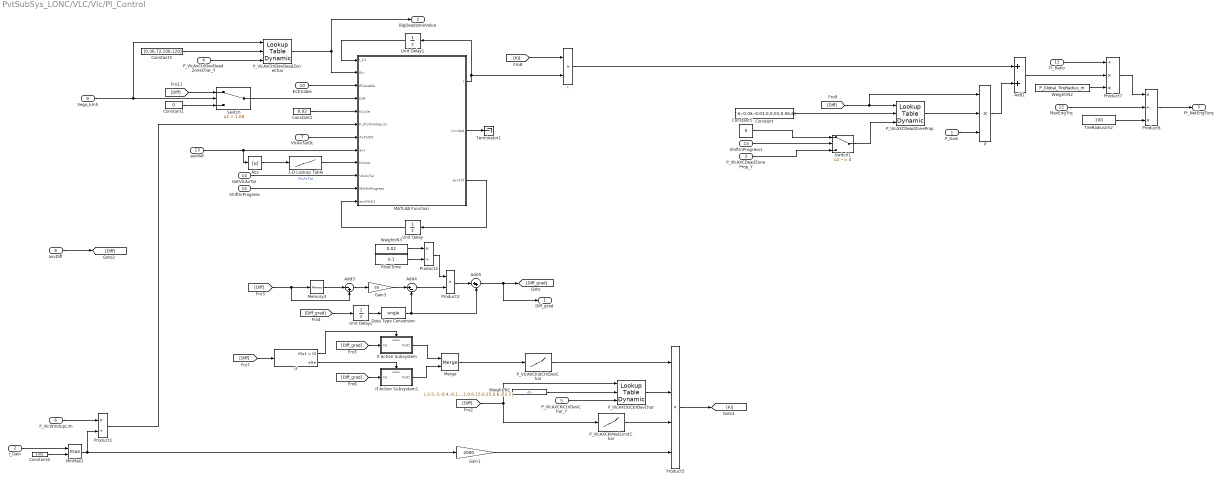
== system PvtSubSys_LONC/VLC/Vlc/PI_Control ==
  P_Gain : Inport
  I_Gain : Inport  Port=2
  P_VlcAXCDeadZoneProp_Y : Inport  Port=3
  P_VlcAxCtrlDevDeadZoneChar_Y : Inport  Port=4
  P_VlcAXCKiCtrlDevChar_Y : Inport  Port=5
  P_VlcWindupLim : Inport  Port=6
  VlcAxTarDt : Inport  Port=7
  axvDiff : Inport  Port=8
  Vego_kmh : Inport  Port=9
  ECEnable : Inport  Port=10
  Tr_Ratio : Inport  Port=11
  MaxEngTrq : Inport  Port=12
  axvRef : Inport  Port=13
  GetVlcAxTar : Inport  Port=14
  ShiftInProgress : Inport  Port=15
  1-D Lookup Table : Lookup_n-D  NumberOfTableDimensions=1  BreakpointsForDimension1=[0,0.01,0.05,0.1,0.2,0.5]  Table=[0.02,0.06,0.1,0.2,0.3,0.3]  InternalRulePriority=Speed  RndMeth=Simplest  InputSameDT=on
  Abs : Abs
  Add1 : Sum
  Add3 : Sum  Inputs=|-+
  Add4 : Sum  Inputs=|+-  AccumDataTypeStr=single
  Add5 : Sum  Inputs=|++  AccumDataTypeStr=single
  Constant : Constant  Value=[-6,-0.06,-0.03,0,0.03,0.06,6]  OutDataTypeStr=single
  Constant1 : Constant  Value=0  OutDataTypeStr=single
  Constant2 : Constant  Value=0.02  OutDataTypeStr=single
  Constant3 : Constant  Value=[0,36,72,108,120]  OutDataTypeStr=single
  Constant4 : Constant  Value=0.001  OutDataTypeStr=single
  Constant5 : Constant  Value=0  OutDataTypeStr=single
  Data Type Conversion : DataTypeConversion  OutDataTypeStr=single
  FilterTime : Constant  Value=0.1  OutDataTypeStr=single
  Gain1 : Gain  Gain=2000
  Gain3 : Gain  Gain=50
  I : Product  RndMeth=Zero
  If : If
  If Action Subsystem : Subsystem  TreatAsAtomicUnit=on
  If Action Subsystem1 : Subsystem  TreatAsAtomicUnit=on
  MATLAB Function : MATLAB Function  TreatAsAtomicUnit=on
  Memory3 : Memory  InheritSampleTime=on
  Merge : Merge
  MinMax1 : MinMax  Function=max  Inputs=2
  P : Product  Inputs=3  RndMeth=Zero
  P_VlcAXCDeadZoneProp : simulink/Lookup Tables/Lookup Table Dynamic  LookUpMeth=Interpolation-Use End Values  OutDataType=fixdt('single')  OutScaling=[]  OutputDataTypeScalingMode=Specify via dialog  OutDataTypeStr=single  DoSatur=off
  P_VlcAXCKiCtrlDevChar : simulink/Lookup Tables/Lookup Table Dynamic  LookUpMeth=Interpolation-Use End Values  OutDataType=fixdt('single')  OutScaling=[]  OutputDataTypeScalingMode=Specify via dialog  OutDataTypeStr=single  DoSatur=off
  P_VlcAXCKiModLimitChar : Lookup_n-D  NumberOfTableDimensions=1  BreakpointsForDimension1=[-2,-0.9,-0.5,1.5,7,10]  Table=[0,0,1,1,0,0]  RndMeth=Simplest  InputSameDT=on
  P_VlcAXCKidCtrlDevChar : Lookup_n-D  NumberOfTableDimensions=1  BreakpointsForDimension1=[-6,-1.3,-0.2,0.3,2.5,15]  Table=[0.25,0.55,0.9,1.1,1.15,1.3]  RndMeth=Simplest  InputSameDT=on
  P_VlcAxCtrlDevDeadZoneChar : simulink/Lookup Tables/Lookup Table Dynamic  LookUpMeth=Interpolation-Use End Values  OutDataType=fixdt('single')  OutScaling=[]  OutputDataTypeScalingMode=Specify via dialog  OutDataTypeStr=single  DoSatur=off
  Product1 : Product  Inputs=*/  RndMeth=Zero
  Product3 : Product  Inputs=**  RndMeth=Zero
  Product4 : Product  Inputs=*/  RndMeth=Zero
  Product5 : Product  Inputs=4  RndMeth=Zero
  Product7 : Product  Inputs=/**  RndMeth=Zero
  Product8 : Product  Inputs=*/*  RndMeth=Zero
  ShiftInProgress1 : InportShadow  Port=15
  Switch : Switch  Criteria=u2 > Threshold  Threshold=1.08
  Switch1 : Switch  Criteria=u2 ~= 0
  Terminator1 : Terminator
  TireRadius/m2 : Constant  Value=100  OutDataTypeStr=single
  Unit Delay : UnitDelay  SampleTime=-1  HasFrameUpgradeWarning=on
  Unit Delay1 : UnitDelay  SampleTime=-1  HasFrameUpgradeWarning=on
  Unit Delay2 : UnitDelay  InitialCondition=single(0)  SampleTime=-1  HasFrameUpgradeWarning=on
  Weight/N1 : Constant  Value=[-2.5,-2,-0.4,-0.17,-0.1,0,0.15,0.25,0.6,3,3.5]  OutDataTypeStr=single
  Weight/N2 : Constant  Value=P_Global_TireRadius_m
  Weight/N3 : Constant  Value=0.02  OutDataTypeStr=single
  Diff_grad : Outport
  BigDeadzoneValue : Outport  Port=2
  PI_NetEngTorq : Outport  Port=3
  wires:
  Data Type Conversion/1 -> Add4/2, Add5/2
  Switch1/1 -> P_VlcAXCDeadZoneProp/3
  Constant5/1 -> Switch1/1
  ShiftInProgress1/1 -> Switch1/2
  Unit Delay/1 -> MATLAB Function/12(axvFiltK1)
  GetVlcAxTar/1 -> MATLAB Function/10(VlcAxTar)  "VlcAxTar"
  axvRef/1 -> Abs/1, MATLAB Function/8(axv)
  ShiftInProgress/1 -> MATLAB Function/11(ShiftInProgress)
  Abs/1 -> 1-D Lookup Table/1
  1-D Lookup Table/1 -> MATLAB Function/9(tConst)
  I_Gain/1 -> MinMax1/1
  Constant4/1 -> MinMax1/2
  axvDiff/1 -> [Diff]
  MATLAB Function/2(Limited) -> Terminator1/1
  Gain1/1 -> Product5/4
  Constant/1 -> P_VlcAXCDeadZoneProp/2
  MATLAB Function/3(axvFilt) -> Unit Delay/1
  Product1/1 -> MATLAB Function/6(P_VlcWindupLim)
  MinMax1/1 -> Product1/2, Gain1/1
  VlcAxTarDt/1 -> MATLAB Function/7(AxTarDt)
  P_VlcWindupLim/1 -> Product1/1
  I/1 -> Add1/1
  P_VlcAXCKiCtrlDevChar_Y/1 -> P_VlcAXCKiCtrlDevChar/3
  Weight/N1/1 -> P_VlcAXCKiCtrlDevChar/2
  Add1/1 -> Product7/2
  Product8/1 -> PI_NetEngTorq/1
  Weight/N2/1 -> Product7/3
  Tr_Ratio/1 -> Product7/1
  Product7/1 -> Product8/1
  MaxEngTrq/1 -> Product8/2
  TireRadius/m2/1 -> Product8/3
  P_VlcAxCtrlDevDeadZoneChar/1 -> MATLAB Function/2(Err), BigDeadzoneValue/1
  P_VlcAxCtrlDevDeadZoneChar_Y/1 -> P_VlcAxCtrlDevDeadZoneChar/3
  Constant3/1 -> P_VlcAxCtrlDevDeadZoneChar/2
  Unit Delay1/1 -> MATLAB Function/1(I_k1)
  ECEnable/1 -> MATLAB Function/3(ECenable)
  Switch/1 -> MATLAB Function/4(Diff)
  Constant2/1 -> MATLAB Function/5(tCycle)
  P_VlcAXCDeadZoneProp_Y/1 -> Switch1/3
  P_VlcAXCDeadZoneProp/1 -> P/2
  MATLAB Function/1(I) -> I/2, Unit Delay1/1
  [Diff] -> P_VlcAXCDeadZoneProp/1, P/1
  Product5/1 -> [Ki]
  P_VlcAXCKiModLimitChar/1 -> Product5/3
  P_VlcAXCKiCtrlDevChar/1 -> Product5/2
  P_VlcAXCKidCtrlDevChar/1 -> Product5/1
  [Diff] -> P_VlcAXCKiModLimitChar/1, P_VlcAXCKiCtrlDevChar/1
  FilterTime/1 -> Product4/2
  Product4/1 -> Product3/1
  Weight/N3/1 -> Product4/1
  [Diff] -> If/1
  Merge/1 -> P_VlcAXCKidCtrlDevChar/1
  If Action Subsystem1/1(Out1) -> Merge/2
  If Action Subsystem/1(Out1) -> Merge/1
  [Diff_grad] -> If Action Subsystem1/1(In1)
  [Diff_grad] -> If Action Subsystem/1(In1)
  If/2 -> If Action Subsystem1/Action
  If/1 -> If Action Subsystem/Action
  [Diff] -> Add3/2, Memory3/1
  Gain3/1 -> Add4/1
  Add5/1 -> [Diff_grad], Diff_grad/1
  Product3/1 -> Add5/1
  Add4/1 -> Product3/2
  Add3/1 -> Gain3/1
  Unit Delay2/1 -> Data Type Conversion/1
  [Diff_grad] -> Unit Delay2/1
  Memory3/1 -> Add3/1
  Constant1/1 -> Switch/3
  Vego_kmh/1 -> Switch/2, P_VlcAxCtrlDevDeadZoneChar/1
  [Diff] -> Switch/1
  [Ki] -> I/1
  P/1 -> Add1/2
  P_Gain/1 -> P/3

== system PvtSubSys_LONC/VLC/Vlc/Subsystem ==
  u : Inport
  MATLAB Function : MATLAB Function  TreatAsAtomicUnit=on
  Memory5 : Memory  InheritSampleTime=on
  Tapped Delay2 : simulink/Discrete/Tapped Delay  vinit=0.0  samptime=-1  NumDelays=1  DelayOrder=Newest  includeCurrent=on
  ACCModeSts : Outport
  wires:
  MATLAB Function/1(ACCModeSts) -> ACCModeSts/1
  u/1 -> Tapped Delay2/1
  Tapped Delay2/1 -> MATLAB Function/1(u)
  MATLAB Function/2(CounterK1) -> Memory5/1
  Memory5/1 -> MATLAB Function/2(Counter)
